simulink model "Use_Cases_N2_b"  (R2020b)
settings: Solver=ode3  StartTime=0.0  StopTime=inf  FixedStep=0.05  RelTol=1e-3
libraries: simulink x2, XBotBlockToolbox x1, Utilities x1

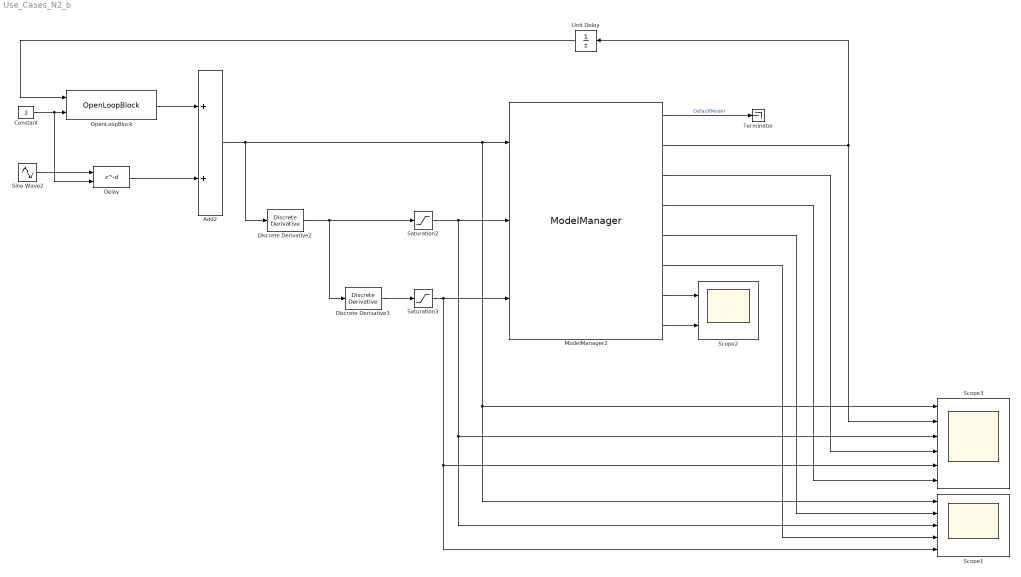
== system Use_Cases_N2_b ==
  Add2 : Sum
  Constant : Constant  Value=2
  Delay : Delay  DelayLengthSource=Input port  DelayLength=1  InitialCondition=0
  Discrete Derivative2 : simulink/Discrete/Discrete Derivative  gainval=1.0  ICPrevScaledInput=0.0  OutMin=[]  OutMax=[]  OutDataType=fixdt(1, 16)  OutScaling=2^-10  DoSatur=off
  Discrete Derivative3 : simulink/Discrete/Discrete Derivative  gainval=1.0  ICPrevScaledInput=0.0  OutMin=[]  OutMax=[]  OutDataType=fixdt(1, 16)  OutScaling=2^-10  DoSatur=off
  ModelManager2 : XBotBlockToolbox/ModelManager  ModelName=DefaultModel  RobotName=DefaultRobot  UseExtModel=Off  SyncWithRobot=Off  GetFloatingBaseList={}  SetFloatingBaseComponent=Off  GravityRequest=Off  ReadingsList={ 'qJ', 'qJdot', 'qJddot', 'qJ_ref', 'qJdot_ref' }  MechanicalLimitsList={}  MechanicalLimitsCheck=On  MechanicalLimitsEnforce=On  SensorList={}  ReferencesList={ 'qJ_ref', 'qJdot_ref', 'qJddot_ref' }  OldModelName=DefaultModel
  OpenLoopBlock : Utilities/OpenLoopBlock  SystemSampleTime=-1  VariantActivationTime=update diagram  Latency=0  AutoFrameSizeCalculation=off
  Saturation2 : Saturate  UpperLimit=0.2  LowerLimit=-0.2
  Saturation3 : Saturate  UpperLimit=0.2  LowerLimit=-0.2
  Scope1 : Scope  NumInputPorts=5
  Scope2 : Scope  NumInputPorts=2
  Scope3 : Scope  NumInputPorts=6
  Sine Wave2 : Sin  Amplitude=0.2  SampleTime=0
  Terminator : Terminator
  Unit Delay : UnitDelay  SampleTime=-1  HasFrameUpgradeWarning=on
  wires:
  ModelManager2/2 -> Scope3/2, Unit Delay/1
  ModelManager2/1 -> Terminator/1  "DefaultModel"
  ModelManager2/4 -> Scope3/6
  ModelManager2/5 -> Scope1/2
  Constant/1 -> Delay/2, OpenLoopBlock/2
  ModelManager2/7 -> Scope2/1
  ModelManager2/8 -> Scope2/2
  Add2/1 -> Discrete Derivative2/1, Scope3/1, Scope1/1, ModelManager2/1
  Discrete Derivative2/1 -> Discrete Derivative3/1, Saturation2/1
  Saturation2/1 -> Scope3/3, Scope1/3, ModelManager2/2
  Discrete Derivative3/1 -> Saturation3/1
  Saturation3/1 -> Scope1/5, Scope3/5, ModelManager2/3
  Unit Delay/1 -> OpenLoopBlock/1
  ModelManager2/3 -> Scope3/4
  ModelManager2/6 -> Scope1/4
  OpenLoopBlock/1 -> Add2/1
  Sine Wave2/1 -> Delay/1
  Delay/1 -> Add2/2
